simulink subsystem "force_to_pwm"  (R2025b)
settings: Solver=VariableStepAuto  StartTime=0.0  StopTime=10.0  RelTol=1e-3
undefined symbols (not defined in the file or in its folder): ccw_force, ccw_pwm, cw_force, cw_pwm, dt_control, pwm_lower_limit, pwm_upper_limit, voltage
settings Model: Creator=koryh  LastModifiedBy=koryh

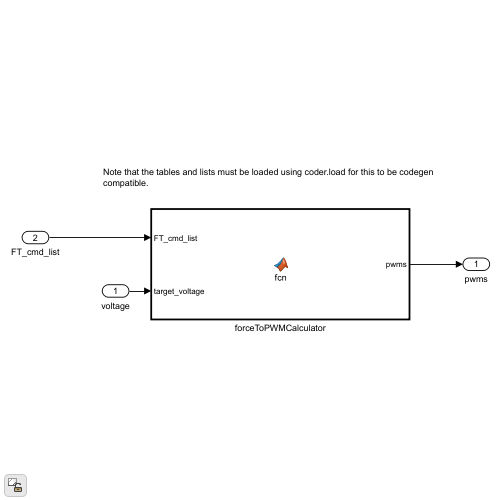
[thumbnail: Simulink's stored preview of the top-level diagram]
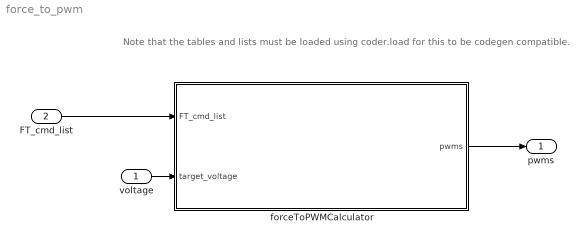
== system force_to_pwm ==
  note: Note that the tables and lists must be loaded using coder.load for this to be codegen compatible.
  voltage : Inport
  FT_cmd_list : Inport  Port=2  PortDimensions=[8,1]  SampleTime=dt_control
  forceToPWMCalculator : MATLAB Function  TreatAsAtomicUnit=on
  pwms : Outport
  wires:
  voltage/1 -> forceToPWMCalculator/2(target_voltage)
  forceToPWMCalculator/1(pwms) -> pwms/1
  FT_cmd_list/1 -> forceToPWMCalculator/1(FT_cmd_list)

== matlab function force_to_pwm/forceToPWMCalculator ==
  data: FT_cmd_list input; target_voltage input; pwms output; cw_pwm parameter; ccw_pwm parameter; cw_force parameter; ccw_force parameter; voltage parameter; pwm_upper_limit parameter; pwm_lower_limit parameter
function pwms = fcn(FT_cmd_list, target_voltage, cw_pwm, ccw_pwm, cw_force, ccw_force, voltage, pwm_upper_limit, pwm_lower_limit)

pwms = forceToPWMCalculator(FT_cmd_list, target_voltage, cw_pwm, ccw_pwm, cw_force, ccw_force, voltage, pwm_upper_limit, pwm_lower_limit);
